simulink model "Rate_Meas_RS232_HFC_2P"  (Simulink 7.8)
settings: Solver=VariableStepDiscrete  StartTime=0.0  StopTime=Inf  FixedStep=Ts/4  RelTol=1e-3
PreLoadFcn:
  | clear all;
  | close all;
  | clc;
  | 
  | Ts = 0.01;          % clk (period)
  | Ns =  1;
StartFcn:
  | clc;
  | close all;
  | 
  | Ns =  200;      % Characters to Tx and to Rx
  | minV = 0;       %  minimum data value
  | maxV = 255;       %  minimum data value
  | Tx_array = randi([minV maxV], 1, Ns, 'uint8');
  | Rx_array = randi([minV maxV], 1, Ns, 'uint8');
  | 
  | 
  | disp('Opening the RS232 ports . . . . . ');
  | s1 = serial('COM34','BaudRate',9600,'Parity','none', 'Terminator', '');
  | set(s1, 'FlowControl', 'none');
  | set(s1, 'InputBufferSize', 1);
  | set(s1, 'OutputBufferSize', 1);
  | fopen(s1)
  | s2 = serial('COM57','BaudRate',9600,'Parity','none', 'Terminator', '');
  | set(s2, 'FlowControl', 'none');
  | set(s2, 'InputBufferSize', 1);
  | set(s2, 'OutputBufferSize', 1);
  | fopen(s2)
  | disp('RS232 ports activated');
  | disp(' ');
  | 
  | s1.RequestToSend = 'on';         %  Rx ON
  | s2.RequestToSend = 'on';
  | 
  | b2o_s1 = uint8(0);
  | d2o_s1 = uint8(0);
  | b2r_s1 = uint8(0);
  | d2r_s1 = uint8(0);
  | rts_s1 = uint8(0);
  | cts_s1 = uint8(0);
  | 
  | b2o_s2 = uint8(0);
  | d2o_s2 = uint8(0);
  | b2r_s2 = uint8(0);
  | d2r_s2 = uint8(0);
  | rts_s2 = uint8(0);
  | cts_s2 = uint8(0);
  | 
  | ts = tic;
StopFcn:
  | e_time = toc(ts);
  | 
  | %
  | %   RS232 ports release
  | %
  | disp(' ');
  | disp('Deactivating RS232 ports ......');
  | 
  | fclose(s1)
  | delete(s1)
  | clear s1
  | 
  | fclose(s2)
  | delete(s2)
  | clear s2
  | 
  | fprintf('RS232 ports deactivated\n');
  | 
  | if Tx_array == Rx_array
  |   disp('Data exchange without errors');
  |   fprintf('\nData Rate = %4.2f Bps\n', Ns/e_time);
  | else
  |    Ne = sum((Tx_array - Rx_array) ~= 0);
  |    fprintf('\nData exchange with %d errors in %d data charactes\n\n', Ne, Ns);
  | end
libraries: simulink x1
settings Model: Creator=theodore  LastModifiedBy=theodore
settings DebuggingCC: SolverPrmCheckMsg=none
settings CodeAppCC: CustomSymbolStrType=$N$R$M_T

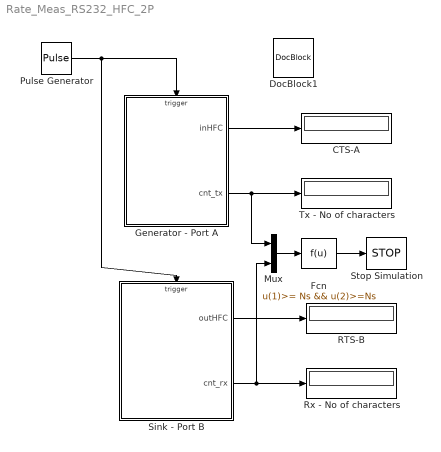
== system Rate_Meas_RS232_HFC_2P ==
  CTS-A : Display
  DocBlock1 : simulink/Model-Wide Utilities/DocBlock  DocumentType=Text
      content=|
      | Generator using RTS  and Sink using CTS
  Fcn : Fcn  Expr=u(1)>= Ns && u(2)>=Ns
  Generator - Port A : Stateflow chart  TreatAsAtomicUnit=on
  Mux : Mux  Inputs=2
  Pulse Generator : DiscretePulseGenerator  PulseType=Time based  Period=Ts  PulseWidth=50
  RTS-B : Display
  Rx - No of characters : Display
  Sink - Port B : Stateflow chart  TreatAsAtomicUnit=on
  Stop Simulation : Stop
  Tx - No of characters : Display
  wires:
  Pulse Generator/1 -> Generator - Port A/Trigger, Sink - Port B/Trigger
  Sink - Port B/2(cnt_rx) -> Rx - No of characters/1, Mux/2
  Sink - Port B/1(outHFC) -> RTS-B/1
  Generator - Port A/1(inHFC) -> CTS-A/1
  Generator - Port A/2(cnt_tx) -> Tx - No of characters/1, Mux/1
  Fcn/1 -> Stop Simulation/1
  Mux/1 -> Fcn/1

== stateflow chart Sink - Port B ==
  state RxState
    en: ml('DIn_2');
    Val_rx = ml.d2r_s2;
    cnt_rx = cnt_rx + 1;
    ml.Rx_array[cnt_rx] = Val_rx;
  state IniState
  IniState -> (junction 5) : {ml('B2R_2'); }
  RxState -> IniState
  (default) -> IniState : {cnt_rx = 0;
      | ml.rts_s2 = 1;
      | ml('CTS_2');
      | outHFC = 1;
      | ml('RTS_2');}
  (junction 5) -> IniState [order 1] : [ml.b2r_s2 == 0 ]
  (junction 5) -> RxState [order 2]
  data: outHFC output double =1; Val_rx local uint8; cnt_rx output double
  events: CLK input RISING_EDGE_EVENT

== stateflow chart Generator - Port A ==
  state Dcalc
    en: ml('CTS_1');
    LBstatus_tx = ml.cts_s1;
    inHFC = LBstatus_tx;
  state IniState
    ml('CTS_1');
    LBstatus_tx = ml.cts_s1;
    inHFC = LBstatus_tx;
  state TxState
    en: cnt_tx = cnt_tx + 1;
    Val_tx = ml.Tx_array[cnt_tx];
    ml.d2o_s1 = Val_tx;
    ml('DOut_1');
  state Idle
  (junction 22) -> TxState [order 1] : [LBstatus_tx  ~= 0 ]
  (junction 21) -> Dcalc [order 2]
  (default) -> IniState : {cnt_tx = 0;}
  (junction 21) -> IniState [order 1] : [ml.b2o_s1 > 0 || LBstatus_tx == 0]
  TxState -> (junction 23)
  IniState -> (junction 21) : {ml('B2O_1'); }
  Dcalc -> (junction 22)
  (junction 22) -> Dcalc [order 2]
  (junction 23) -> Idle [order 1] : [cnt_tx == ml.Ns]
  (junction 23) -> IniState [order 2]
  data: inHFC output double; cnt_tx output double; Val_tx local uint8; LBstatus_tx local double =0
  events: CLK input RISING_EDGE_EVENT
